simulink model "CarSim_SCANeR_UDP_LKA_THESIS"  (R2019a)
settings: Solver=FixedStepDiscrete  StartTime=0.0  StopTime=inf  FixedStep=0.001  RelTol=1e-3  EnableMultiTasking=on
undefined symbols (not defined in the file or in its folder): DiscIntNeverNeededParam
libraries: simulink x11, xpcutilitieslib x2, xpcrtudplib x2, dspnetwork x1
(part 1 of 2)
settings Model: ExtModeTrigDuration=10000  Creator=llacroix  LastModifiedBy=wilkerson.102
settings SolverCC: PositivePriorityOrder=on  InsertRTBMode=Always
settings DataIOCC: ReturnWorkspaceOutputs=off
settings OptimizationCC: UseFloatMulNetSlope=on
settings DebuggingCC: ArithmeticOperatorsInVariantConditions=warning
settings SFSimCC: SimUseLocalCustomCode=off
settings RTWCC: Description=Generic Real-Time Target  RTWUseLocalCustomCode=off  TargetLang=C++
settings CodeAppCC: StateflowObjectComments=on
settings GRTTargetCC: TargetLangStandard=C++03 (ISO)  MatFileLogging=off  MultiInstanceERTCode=on  CodeInterfacePackaging=C++ class

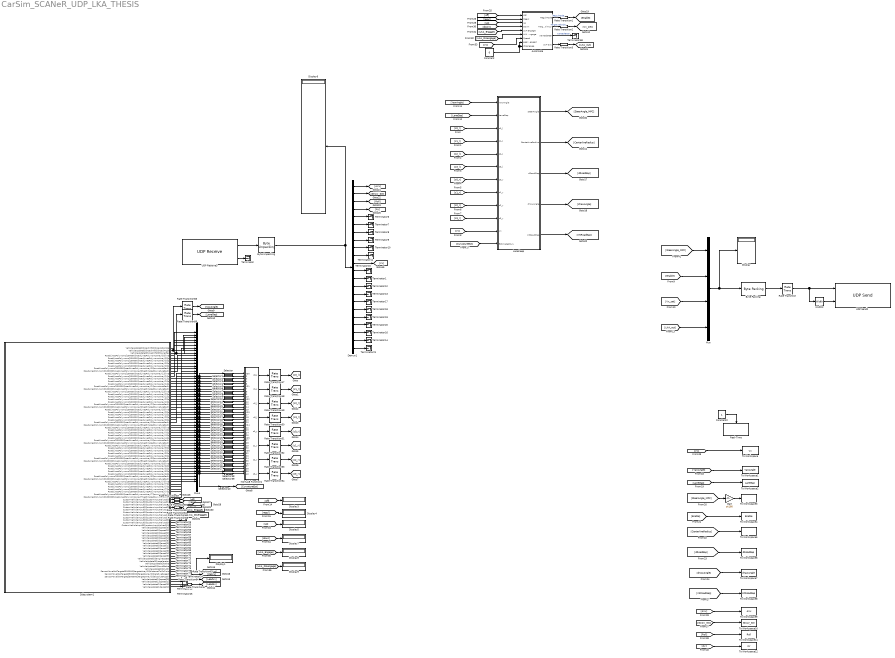
== system CarSim_SCANeR_UDP_LKA_THESIS ==
  Automate : Subsystem
  "Byte Packing " : xpcutilitieslib/Byte Packing   MaskPackedDataType=uint8  MaskUnpackedDataTypes={'double'}  MaskAlignment=1
  "Byte Unpacking " : xpcutilitieslib/Byte Unpacking   MaskUnpackedDataTypes={'double'}  MaskUnpackedDataSizes={[22]}  MaskAlignment=1
      settings: SourceProductName=Simulink Real-Time  SourceProductBaseCode=XP
  Constant : Constant  Value=0
  Constant2 : Constant
  Demux1 : Demux  Outputs=22
  Display{,1,3..9} (9 alike) : Display
  Gain : Gain  Gain=pi/180
  LaneKeep : Subsystem
  MATLAB Function1 : Subsystem
      mask help: Simulink:masks:GenSFuncDesc_MD
      mask Help: eval('feval(''rtwprivate'',''rtwhelpview'',''rtw_sfcn_block'')');
  Mux : Mux
  Mux4 : Mux  Inputs=59
  Rate Transition{,1..3,5,47..64} (23 alike) : RateTransition
  Real-Time : Subsystem
  Selector : Selector  InputPortWidth=59  IndexOptions=Index vector (dialog)  Indices=4  OutputSizes=1
  Selector1 : Selector  InputPortWidth=59  IndexOptions=Index vector (dialog)  Indices=5  OutputSizes=1
  Selector10 : Selector  InputPortWidth=59  IndexOptions=Index vector (dialog)  Indices=18  OutputSizes=1
  Selector11 : Selector  InputPortWidth=59  IndexOptions=Index vector (dialog)  Indices=19  OutputSizes=1
  Selector12 : Selector  InputPortWidth=59  IndexOptions=Index vector (dialog)  Indices=20  OutputSizes=1
  Selector13 : Selector  InputPortWidth=59  IndexOptions=Index vector (dialog)  Indices=21  OutputSizes=1
  Selector14 : Selector  InputPortWidth=59  IndexOptions=Index vector (dialog)  Indices=22  OutputSizes=1
  Selector15 : Selector  InputPortWidth=59  IndexOptions=Index vector (dialog)  Indices=25  OutputSizes=1
  Selector16 : Selector  InputPortWidth=59  IndexOptions=Index vector (dialog)  Indices=26  OutputSizes=1
  Selector17 : Selector  InputPortWidth=59  IndexOptions=Index vector (dialog)  Indices=27  OutputSizes=1
  Selector18 : Selector  InputPortWidth=59  IndexOptions=Index vector (dialog)  Indices=28  OutputSizes=1
  Selector19 : Selector  InputPortWidth=59  IndexOptions=Index vector (dialog)  Indices=29  OutputSizes=1
  Selector2 : Selector  InputPortWidth=59  IndexOptions=Index vector (dialog)  Indices=6  OutputSizes=1
  Selector20 : Selector  InputPortWidth=59  IndexOptions=Index vector (dialog)  Indices=32  OutputSizes=1
  Selector21 : Selector  InputPortWidth=59  IndexOptions=Index vector (dialog)  Indices=33  OutputSizes=1
  Selector22 : Selector  InputPortWidth=59  IndexOptions=Index vector (dialog)  Indices=34  OutputSizes=1
  Selector23 : Selector  InputPortWidth=59  IndexOptions=Index vector (dialog)  Indices=35  OutputSizes=1
  Selector24 : Selector  InputPortWidth=59  IndexOptions=Index vector (dialog)  Indices=36  OutputSizes=1
  Selector25 : Selector  InputPortWidth=59  IndexOptions=Index vector (dialog)  Indices=39  OutputSizes=1
  Selector26 : Selector  InputPortWidth=59  IndexOptions=Index vector (dialog)  Indices=40  OutputSizes=1
  Selector27 : Selector  InputPortWidth=59  IndexOptions=Index vector (dialog)  Indices=41  OutputSizes=1
  Selector28 : Selector  InputPortWidth=59  IndexOptions=Index vector (dialog)  Indices=42  OutputSizes=1
  Selector29 : Selector  InputPortWidth=59  IndexOptions=Index vector (dialog)  Indices=43  OutputSizes=1
  Selector3 : Selector  InputPortWidth=59  IndexOptions=Index vector (dialog)  Indices=7  OutputSizes=1
  Selector30 : Selector  InputPortWidth=59  IndexOptions=Index vector (dialog)  Indices=46  OutputSizes=1
  Selector31 : Selector  InputPortWidth=59  IndexOptions=Index vector (dialog)  Indices=47  OutputSizes=1
  Selector32 : Selector  InputPortWidth=59  IndexOptions=Index vector (dialog)  Indices=48  OutputSizes=1
  Selector33 : Selector  InputPortWidth=59  IndexOptions=Index vector (dialog)  Indices=49  OutputSizes=1
  Selector34 : Selector  InputPortWidth=59  IndexOptions=Index vector (dialog)  Indices=50  OutputSizes=1
  Selector35 : Selector  InputPortWidth=59  IndexOptions=Index vector (dialog)  Indices=53  OutputSizes=1
  Selector36 : Selector  InputPortWidth=59  IndexOptions=Index vector (dialog)  Indices=54  OutputSizes=1
  Selector37 : Selector  InputPortWidth=59  IndexOptions=Index vector (dialog)  Indices=55  OutputSizes=1
  Selector38 : Selector  InputPortWidth=59  IndexOptions=Index vector (dialog)  Indices=56  OutputSizes=1
  Selector39 : Selector  InputPortWidth=59  IndexOptions=Index vector (dialog)  Indices=57  OutputSizes=1
  Selector4 : Selector  InputPortWidth=59  IndexOptions=Index vector (dialog)  Indices=8  OutputSizes=1
  Selector40 : Selector  InputPortWidth=59  IndexOptions=Index vector (dialog)  Indices=10  OutputSizes=1
  Selector5 : Selector  InputPortWidth=59  IndexOptions=Index vector (dialog)  Indices=11  OutputSizes=1
  Selector6 : Selector  InputPortWidth=59  IndexOptions=Index vector (dialog)  Indices=12  OutputSizes=1
  Selector7 : Selector  InputPortWidth=59  IndexOptions=Index vector (dialog)  Indices=13  OutputSizes=1
  Selector8 : Selector  InputPortWidth=59  IndexOptions=Index vector (dialog)  Indices=14  OutputSizes=1
  Selector9 : Selector  InputPortWidth=59  IndexOptions=Index vector (dialog)  Indices=15  OutputSizes=1
  Subsystem1 : Subsystem
  Terminator{,1,6..25,53..63,68..78} (44 alike) : Terminator
  To Workspace : ToWorkspace  VariableName=Vx  SampleTime=-1
      settings: Save2DSignal=2-D array (concatenate along first dimension)
  To Workspace1 : ToWorkspace  VariableName=YawAngle  SampleTime=-1
      settings: Save2DSignal=2-D array (concatenate along first dimension)
  To Workspace10 : ToWorkspace  VariableName=StrAV_SW  SampleTime=-1
      settings: Save2DSignal=2-D array (concatenate along first dimension)
  To Workspace11 : ToWorkspace  VariableName=Roll  SampleTime=-1
      settings: Save2DSignal=2-D array (concatenate along first dimension)
  To Workspace12 : ToWorkspace  VariableName=Ay  SampleTime=-1
      settings: Save2DSignal=2-D array (concatenate along first dimension)
  To Workspace2 : ToWorkspace  VariableName=LaneGap  SampleTime=-1
      settings: Save2DSignal=2-D array (concatenate along first dimension)
  To Workspace3 : ToWorkspace  VariableName=SteerAngle_MPC  SampleTime=-1
      settings: Save2DSignal=2-D array (concatenate along first dimension)
  To Workspace4 : ToWorkspace  VariableName=Enable  SampleTime=-1
      settings: Save2DSignal=2-D array (concatenate along first dimension)
  To Workspace5 : ToWorkspace  VariableName=CenterlineRadius  SampleTime=-1
      settings: Save2DSignal=2-D array (concatenate along first dimension)
  To Workspace6 : ToWorkspace  VariableName=dRoadGap  SampleTime=-1
      settings: Save2DSignal=2-D array (concatenate along first dimension)
  To Workspace7 : ToWorkspace  VariableName=dYawAngle  SampleTime=-1
      settings: Save2DSignal=2-D array (concatenate along first dimension)
  To Workspace8 : ToWorkspace  VariableName=intRoadGap  SampleTime=-1
      settings: Save2DSignal=2-D array (concatenate along first dimension)
  To Workspace9 : ToWorkspace  VariableName=AVx  SampleTime=-1
      settings: Save2DSignal=2-D array (concatenate along first dimension)
  UDP Receive3 : xpcrtudplib/UDP Receive  ipAddressVal=Use host-target connection  localPort=25002  rcvWidth=176  rcvFmAny=off  fmAddress=0.0.0.0  rcvMulticast=off  multicastAddress={}  maxUDPQueue=8  sampleTime=0.001
      settings: SourceProductName=Simulink Real-Time
  UDP Send2 : xpcrtudplib/UDP Send  ipAddressVal=Use host-target connection  localPort=-1  toAddress=255.255.255.255  toPort=25003  sampleTime=0.01
      settings: SourceProductName=Simulink Real-Time  SourceProductBaseCode=XP
  Width2 : Width
  wires:
  Width2/1 -> UDP Send2/2
  UDP Receive3/1 -> "Byte Unpacking "/1
  UDP Receive3/2 -> Terminator/1
  LaneKeep/1(SteerAngle) -> [SteerAngle_MPC]
  [YawAngle] -> LaneKeep/1(YawAngle)
  [LaneGap] -> LaneKeep/2(LaneGap)
  [c0_l] -> LaneKeep/3(c0_l)
  [c1_l] -> LaneKeep/4(c1_l)
  [c2_l] -> LaneKeep/5(c2_l)
  [c3_l] -> LaneKeep/6(c3_l)
  [c0_r] -> LaneKeep/7(c0_r)
  [c1_r] -> LaneKeep/8(c1_r)
  [c2_r] -> LaneKeep/9(c2_r)
  [c3_r] -> LaneKeep/10(c3_r)
  [Vx] -> LaneKeep/11(Vx)
  Demux1/11 -> [Vx]
  Demux1/13 -> Terminator1/1
  [SteerAngle_MPC] -> Mux/1
  "Byte Unpacking "/1 -> Demux1/1, Display6/1
  Mux/1 -> "Byte Packing "/1, Display/1
  "Byte Packing "/1 -> Rate Transition/1
  Rate Transition64/1 -> [RelVx]
  Rate Transition63/1 -> Display1/1, [RelDist]
  Rate Transition58/1 -> [LKA_Disengage]
  Subsystem1/65(CustomVehicleInput[0]/customInputValues[5]) -> Rate Transition58/1
  Rate Transition62/1 -> [LKA_Engage]
  Subsystem1/64(CustomVehicleInput[0]/customInputValues[4]) -> Rate Transition62/1
  Rate Transition61/1 -> [down]
  Subsystem1/63(CustomVehicleInput[0]/customInputValues[3]) -> Rate Transition61/1
  Rate Transition60/1 -> [up]
  Subsystem1/62(CustomVehicleInput[0]/customInputValues[2]) -> Rate Transition60/1
  Rate Transition59/1 -> [regul]
  Subsystem1/61(CustomVehicleInput[0]/customInputValues[1]) -> Rate Transition59/1
  Subsystem1/60(CustomVehicleInput[0]/customInputValues[0]) -> Rate Transition57/1
  Rate Transition57/1 -> [off]
  Rate Transition56/1 -> [LaneGap]
  Rate Transition55/1 -> [YawAngle]
  Rate Transition54/1 -> [c3_r]
  Rate Transition53/1 -> [c2_r]
  Rate Transition52/1 -> [c1_r]
  Rate Transition51/1 -> [c0_r]
  Rate Transition50/1 -> [c3_l]
  Rate Transition49/1 -> [c2_l]
  Rate Transition48/1 -> [c1_l]
  Rate Transition47/1 -> [c0_l]
  Subsystem1/87(VehicleUpdate[0]/clutch) -> Terminator78/1
  Subsystem1/86(VehicleUpdate[0]/handBrake) -> Terminator77/1
  Subsystem1/85(VehicleUpdate[0]/brake) -> Terminator76/1
  Subsystem1/84(VehicleUpdate[0]/accelerator) -> Terminator75/1
  Subsystem1/83(VehicleUpdate[0]/engineSpeed) -> Terminator74/1
  Subsystem1/82(VehicleUpdate[0]/accel[5]) -> Terminator73/1
  Subsystem1/81(VehicleUpdate[0]/accel[4]) -> Terminator72/1
  Subsystem1/80(VehicleUpdate[0]/accel[3]) -> Terminator71/1
  Subsystem1/79(VehicleUpdate[0]/accel[2]) -> Terminator70/1
  Subsystem1/78(VehicleUpdate[0]/accel[1]) -> Terminator69/1
  Subsystem1/77(VehicleUpdate[0]/accel[0]) -> Terminator63/1
  Subsystem1/76(VehicleUpdate[0]/speed[5]) -> Terminator62/1
  Subsystem1/75(VehicleUpdate[0]/speed[4]) -> Terminator61/1
  Subsystem1/74(VehicleUpdate[0]/speed[3]) -> Terminator60/1
  Subsystem1/73(VehicleUpdate[0]/speed[2]) -> Terminator59/1
  Subsystem1/72(VehicleUpdate[0]/speed[1]) -> Terminator58/1
  Subsystem1/71(VehicleUpdate[0]/speed[0]) -> Terminator57/1
  Subsystem1/70(CustomVehicleInput[0]/customInputValues[10]) -> Terminator56/1
  Subsystem1/69(CustomVehicleInput[0]/customInputValues[9]) -> Terminator55/1
  Subsystem1/68(CustomVehicleInput[0]/customInputValues[8]) -> Terminator54/1
  Subsystem1/67(CustomVehicleInput[0]/customInputValues[7]) -> Terminator53/1
  Subsystem1/66(CustomVehicleInput[0]/customInputValues[6]) -> Terminator23/1
  Subsystem1/59(RoadLinesPolynoms[100000]/roadLinesPolynomsArray[7]/estimatedCurvatureRadius) -> Mux4/59
  Subsystem1/58(RoadLinesPolynoms[100000]/roadLinesPolynomsArray[7]/curvatureRadius) -> Mux4/58
  Subsystem1/57(RoadLinesPolynoms[100000]/roadLinesPolynomsArray[7]/c3) -> Mux4/57
  Subsystem1/56(RoadLinesPolynoms[100000]/roadLinesPolynomsArray[7]/c2) -> Mux4/56
  Subsystem1/55(RoadLinesPolynoms[100000]/roadLinesPolynomsArray[7]/c1) -> Mux4/55
  Subsystem1/54(RoadLinesPolynoms[100000]/roadLinesPolynomsArray[7]/c0) -> Mux4/54
  Subsystem1/53(RoadLinesPolynoms[100000]/roadLinesPolynomsArray[7]/lineId) -> Mux4/53
  Subsystem1/52(RoadLinesPolynoms[100000]/roadLinesPolynomsArray[6]/estimatedCurvatureRadius) -> Mux4/52
  Subsystem1/51(RoadLinesPolynoms[100000]/roadLinesPolynomsArray[6]/curvatureRadius) -> Mux4/51
  Subsystem1/50(RoadLinesPolynoms[100000]/roadLinesPolynomsArray[6]/c3) -> Mux4/50
  Subsystem1/49(RoadLinesPolynoms[100000]/roadLinesPolynomsArray[6]/c2) -> Mux4/49
  Subsystem1/48(RoadLinesPolynoms[100000]/roadLinesPolynomsArray[6]/c1) -> Mux4/48
  Subsystem1/47(RoadLinesPolynoms[100000]/roadLinesPolynomsArray[6]/c0) -> Mux4/47
  Subsystem1/46(RoadLinesPolynoms[100000]/roadLinesPolynomsArray[6]/lineId) -> Mux4/46
  Subsystem1/45(RoadLinesPolynoms[100000]/roadLinesPolynomsArray[5]/estimatedCurvatureRadius) -> Mux4/45
  Subsystem1/44(RoadLinesPolynoms[100000]/roadLinesPolynomsArray[5]/curvatureRadius) -> Mux4/44
  Subsystem1/43(RoadLinesPolynoms[100000]/roadLinesPolynomsArray[5]/c3) -> Mux4/43
  Subsystem1/42(RoadLinesPolynoms[100000]/roadLinesPolynomsArray[5]/c2) -> Mux4/42
  Subsystem1/41(RoadLinesPolynoms[100000]/roadLinesPolynomsArray[5]/c1) -> Mux4/41
  Subsystem1/40(RoadLinesPolynoms[100000]/roadLinesPolynomsArray[5]/c0) -> Mux4/40
  Subsystem1/39(RoadLinesPolynoms[100000]/roadLinesPolynomsArray[5]/lineId) -> Mux4/39
  Subsystem1/38(RoadLinesPolynoms[100000]/roadLinesPolynomsArray[4]/estimatedCurvatureRadius) -> Mux4/38
  Subsystem1/37(RoadLinesPolynoms[100000]/roadLinesPolynomsArray[4]/curvatureRadius) -> Mux4/37
  Subsystem1/36(RoadLinesPolynoms[100000]/roadLinesPolynomsArray[4]/c3) -> Mux4/36
  Subsystem1/35(RoadLinesPolynoms[100000]/roadLinesPolynomsArray[4]/c2) -> Mux4/35
  Subsystem1/34(RoadLinesPolynoms[100000]/roadLinesPolynomsArray[4]/c1) -> Mux4/34
  Subsystem1/33(RoadLinesPolynoms[100000]/roadLinesPolynomsArray[4]/c0) -> Mux4/33
  Subsystem1/32(RoadLinesPolynoms[100000]/roadLinesPolynomsArray[4]/lineId) -> Mux4/32
  Subsystem1/31(RoadLinesPolynoms[100000]/roadLinesPolynomsArray[3]/estimatedCurvatureRadius) -> Mux4/31
  Subsystem1/30(RoadLinesPolynoms[100000]/roadLinesPolynomsArray[3]/curvatureRadius) -> Mux4/30
  Subsystem1/29(RoadLinesPolynoms[100000]/roadLinesPolynomsArray[3]/c3) -> Mux4/29
  Subsystem1/28(RoadLinesPolynoms[100000]/roadLinesPolynomsArray[3]/c2) -> Mux4/28
  Subsystem1/27(RoadLinesPolynoms[100000]/roadLinesPolynomsArray[3]/c1) -> Mux4/27
  Subsystem1/26(RoadLinesPolynoms[100000]/roadLinesPolynomsArray[3]/c0) -> Mux4/26
  Subsystem1/25(RoadLinesPolynoms[100000]/roadLinesPolynomsArray[3]/lineId) -> Mux4/25
  Subsystem1/24(RoadLinesPolynoms[100000]/roadLinesPolynomsArray[2]/estimatedCurvatureRadius) -> Mux4/24
  Subsystem1/23(RoadLinesPolynoms[100000]/roadLinesPolynomsArray[2]/curvatureRadius) -> Mux4/23
  Subsystem1/22(RoadLinesPolynoms[100000]/roadLinesPolynomsArray[2]/c3) -> Mux4/22
  Subsystem1/21(RoadLinesPolynoms[100000]/roadLinesPolynomsArray[2]/c2) -> Mux4/21
  Subsystem1/20(RoadLinesPolynoms[100000]/roadLinesPolynomsArray[2]/c1) -> Mux4/20
  Subsystem1/19(RoadLinesPolynoms[100000]/roadLinesPolynomsArray[2]/c0) -> Mux4/19
  Subsystem1/18(RoadLinesPolynoms[100000]/roadLinesPolynomsArray[2]/lineId) -> Mux4/18
  Subsystem1/17(RoadLinesPolynoms[100000]/roadLinesPolynomsArray[1]/estimatedCurvatureRadius) -> Mux4/17
  Subsystem1/16(RoadLinesPolynoms[100000]/roadLinesPolynomsArray[1]/curvatureRadius) -> Mux4/16
  Subsystem1/15(RoadLinesPolynoms[100000]/roadLinesPolynomsArray[1]/c3) -> Mux4/15
  Subsystem1/14(RoadLinesPolynoms[100000]/roadLinesPolynomsArray[1]/c2) -> Mux4/14
  Subsystem1/13(RoadLinesPolynoms[100000]/roadLinesPolynomsArray[1]/c1) -> Mux4/13
  Subsystem1/12(RoadLinesPolynoms[100000]/roadLinesPolynomsArray[1]/c0) -> Mux4/12
  Subsystem1/11(RoadLinesPolynoms[100000]/roadLinesPolynomsArray[1]/lineId) -> Mux4/11
  Subsystem1/10(RoadLinesPolynoms[100000]/roadLinesPolynomsArray[0]/estimatedCurvatureRadius) -> Mux4/10
  Subsystem1/9(RoadLinesPolynoms[100000]/roadLinesPolynomsArray[0]/curvatureRadius) -> Mux4/9
  Subsystem1/8(RoadLinesPolynoms[100000]/roadLinesPolynomsArray[0]/c3) -> Mux4/8
  Subsystem1/7(RoadLinesPolynoms[100000]/roadLinesPolynomsArray[0]/c2) -> Mux4/7
  Subsystem1/6(RoadLinesPolynoms[100000]/roadLinesPolynomsArray[0]/c1) -> Mux4/6
  Subsystem1/5(RoadLinesPolynoms[100000]/roadLinesPolynomsArray[0]/c0) -> Mux4/5
  Subsystem1/4(RoadLinesPolynoms[100000]/roadLinesPolynomsArray[0]/lineId) -> Mux4/4
  Subsystem1/3(VehicleUpdate[0]/roadInfo[0]/laneGap) -> Mux4/3, Rate Transition56/1
  Subsystem1/2(VehicleUpdate[0]/roadInfo[0]/roadAngle) -> Mux4/2, Rate Transition55/1
  Subsystem1/1(VehicleUpdate[0]/roadInfo[0]/roadAbscissa) -> Mux4/1
  Selector39/1 -> MATLAB Function1/40(c3_7)
  Selector38/1 -> MATLAB Function1/39(c2_7)
  Selector37/1 -> MATLAB Function1/38(c1_7)
  Selector36/1 -> MATLAB Function1/37(c0_7)
  Selector35/1 -> MATLAB Function1/36(ID7)
  Selector34/1 -> MATLAB Function1/35(c3_6)
  Selector33/1 -> MATLAB Function1/34(c2_6)
  Selector32/1 -> MATLAB Function1/33(c1_6)
  Selector31/1 -> MATLAB Function1/32(c0_6)
  Selector30/1 -> MATLAB Function1/31(ID6)
  Selector29/1 -> MATLAB Function1/30(c3_5)
  Selector28/1 -> MATLAB Function1/29(c2_5)
  Selector27/1 -> MATLAB Function1/28(c1_5)
  Selector26/1 -> MATLAB Function1/27(c0_5)
  Selector25/1 -> MATLAB Function1/26(ID5)
  Selector24/1 -> MATLAB Function1/25(c3_4)
  Selector23/1 -> MATLAB Function1/24(c2_4)
  Selector22/1 -> MATLAB Function1/23(c1_4)
  Selector21/1 -> MATLAB Function1/22(c0_4)
  Selector20/1 -> MATLAB Function1/21(ID4)
  Selector19/1 -> MATLAB Function1/20(c3_3)
  Selector18/1 -> MATLAB Function1/19(c2_3)
  Selector17/1 -> MATLAB Function1/18(c1_3)
  Selector16/1 -> MATLAB Function1/17(c0_3)
  Selector15/1 -> MATLAB Function1/16(ID3)
  Selector14/1 -> MATLAB Function1/15(c3_2)
  Selector13/1 -> MATLAB Function1/14(c2_2)
  Selector12/1 -> MATLAB Function1/13(c1_2)
  Selector11/1 -> MATLAB Function1/12(c0_2)
  Selector10/1 -> MATLAB Function1/11(ID2)
  Selector9/1 -> MATLAB Function1/10(c3_1)
  Selector8/1 -> MATLAB Function1/9(c2_1)
  Selector7/1 -> MATLAB Function1/8(c1_1)
  Selector6/1 -> MATLAB Function1/7(c0_1)
  Selector5/1 -> MATLAB Function1/6(ID1)
  Selector4/1 -> MATLAB Function1/5(c3_0)
  Selector3/1 -> MATLAB Function1/4(c2_0)
  Selector2/1 -> MATLAB Function1/3(c1_0)
  Selector1/1 -> MATLAB Function1/2(c0_0)
  Selector/1 -> MATLAB Function1/1(ID0)
  MATLAB Function1/8(c3_r) -> Rate Transition54/1
  MATLAB Function1/7(c2_r) -> Rate Transition53/1
  MATLAB Function1/6(c1_r) -> Rate Transition52/1
  MATLAB Function1/5(c0_r) -> Rate Transition51/1
  MATLAB Function1/4(c3_l) -> Rate Transition50/1
  MATLAB Function1/3(c2_l) -> Rate Transition49/1
  MATLAB Function1/2(c1_l) -> Rate Transition48/1
  MATLAB Function1/1(c0_l) -> Rate Transition47/1
  Mux4/1 -> Selector40/1, Selector39/1, Selector38/1, Selector37/1, Selector36/1, Selector35/1, Selector34/1, Selector33/1, Selector32/1, Selector31/1, Selector30/1, Selector29/1, Selector28/1, Selector27/1, Selector26/1, Selector25/1, Selector24/1, Selector23/1, Selector22/1, Selector21/1, Selector20/1, Selector19/1, Selector18/1, Selector17/1, Selector16/1, Selector15/1, Selector14/1, Selector11/1, Selector10/1, Selector9/1, Selector7/1, Selector6/1, Selector5/1, Selector4/1, Selector3/1, Selector2/1, Selector/1, Selector1/1, Selector8/1, Selector12/1, Selector13/1
  Subsystem1/89(SensorMovableTargets[300000]/targetsArray[0]/relativeSpeedX) -> Rate Transition64/1
  Subsystem1/88(SensorMovableTargets[300000]/targetsArray[0]/distanceToCollision) -> Rate Transition63/1
  Demux1/3 -> [Roll]
  Demux1/5 -> Terminator6/1
  Demux1/6 -> Terminator7/1
  Demux1/7 -> Terminator8/1
  Demux1/8 -> Terminator9/1
  Demux1/9 -> Terminator10/1
  Demux1/10 -> Terminator11/1
  Demux1/14 -> Terminator12/1
  Demux1/15 -> Terminator13/1
  Demux1/21 -> Terminator14/1
  Automate/2(Target (m/s)) -> Rate Transition2/1  "Target Velocity"
  Automate/1(RegulMode) -> Rate Transition1/1  "RegulMode"
  Automate/3(wantedGear) -> Terminator68/1  "wantedGear"
  Demux1/12 -> Terminator15/1
  Demux1/20 -> Terminator16/1
  Automate/4(LKA Out) -> Rate Transition3/1
  Rate Transition1/1 -> [Enable]
  Rate Transition2/1 -> [Vx_set]
  Rate Transition3/1 -> [LKA_out]
  [off] -> Automate/1(Off)
  [regul] -> Automate/2(Regul)
  [up] -> Automate/3(Up)
  [down] -> Automate/4(Down)
  [LKA_Engage] -> Automate/5(LKA Engage)
  [LKA_Disengage] -> Automate/6(LKA Disengage)
  [Vx] -> Automate/7(Speed)
  Constant/1 -> Automate/9(disengage), Automate/8(gearEngaged)
  Rate Transition/1 -> Width2/1, UDP Send2/1
  [Enable] -> Mux/2
  [Vx_set] -> Mux/3
  [LKA_out] -> Mux/4
  [off] -> Display3/1
  [regul] -> Display4/1
  [up] -> Display5/1
  [down] -> Display7/1
  [LKA_Engage] -> Display8/1
  [LKA_Disengage] -> Display9/1
  Demux1/16 -> Terminator17/1
  Demux1/17 -> Terminator18/1
  Demux1/18 -> Terminator19/1
  Demux1/19 -> Terminator20/1
  Demux1/22 -> Terminator21/1
  Selector40/1 -> [CurvatureEst]
  [CurvatureEst] -> LaneKeep/12(EstimatedCurv)
  Rate Transition5/1 -> [LeadAx]
  Subsystem1/91(VehicleUpdate[1]/speed[0]) -> [LeadVx]
  Subsystem1/93(VehicleUpdate[1]/accel[0]) -> Rate Transition5/1
  Subsystem1/94(VehicleUpdate[1]/accel[1]) -> Terminator25/1
  Subsystem1/92(VehicleUpdate[1]/speed[1]) -> Terminator22/1
  Subsystem1/90(SensorMovableTargets[300000]/targetsArray[0]/absoluteAccelX) -> Terminator24/1
  Constant2/1 -> Real-Time/Enable
  [Vx] -> To Workspace/1
  LaneKeep/2(CenterLineRadius) -> [CenterlineRadius]
  [SteerAngle_MPC] -> Gain/1
  LaneKeep/3(dRoadGap) -> [dRoadGap]
  LaneKeep/4(dYawAngle) -> [dYawAngle]
  LaneKeep/5(intRoadGap) -> [intRoadGap]
  [YawAngle] -> To Workspace1/1
  [LaneGap] -> To Workspace2/1
  Gain/1 -> To Workspace3/1
  [Enable] -> To Workspace4/1
  [CenterlineRadius] -> To Workspace5/1
  [dRoadGap] -> To Workspace6/1
  [dYawAngle] -> To Workspace7/1
  [intRoadGap] -> To Workspace8/1
  Demux1/1 -> [AVx]
  Demux1/2 -> [StrAV_SW]
  [AVx] -> To Workspace9/1
  [StrAV_SW] -> To Workspace10/1
  [Roll] -> To Workspace11/1
  Demux1/4 -> [Ay]
  [Ay] -> To Workspace12/1

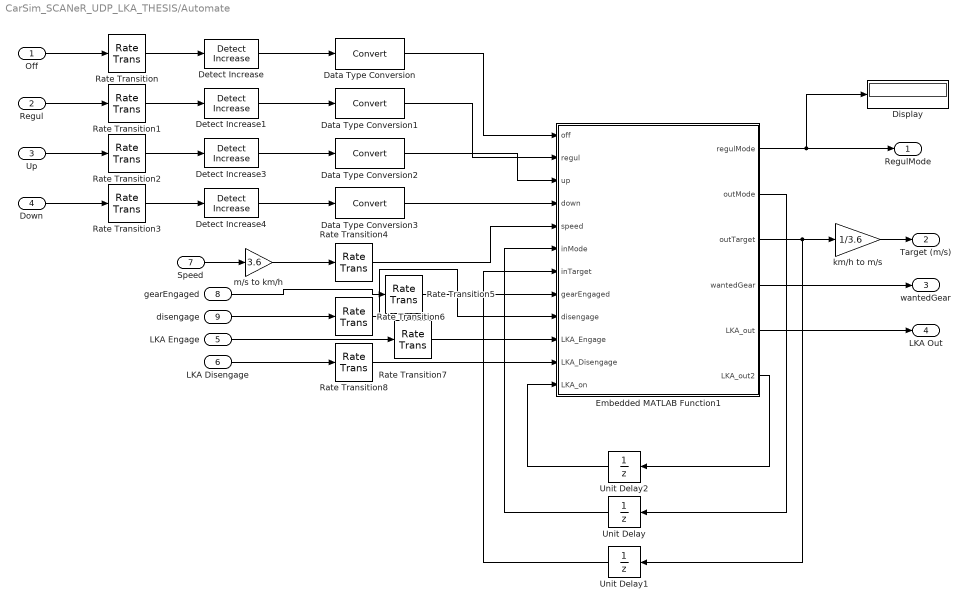
== system CarSim_SCANeR_UDP_LKA_THESIS/Automate ==
  Off : Inport  PortDimensions=1
  Regul : Inport  Port=2  PortDimensions=1
  Up : Inport  Port=3  PortDimensions=1
  Down : Inport  Port=4  PortDimensions=1
  LKA Engage : Inport  Port=5  PortDimensions=1
  LKA Disengage : Inport  Port=6  PortDimensions=1
  Speed : Inport  Port=7  PortDimensions=1
  gearEngaged : Inport  Port=8  PortDimensions=1
  disengage : Inport  Port=9  PortDimensions=1
  Data Type Conversion{,1..3} (4 alike) : DataTypeConversion
  Detect Increase{,1,3..4} (4 alike) : simulink/Logic and Bit Operations/Detect Increase  vinit=0.0  OutDataTypeStr=uint8
  Display : Display
  Embedded MATLAB Function1 : MATLAB Function  TreatAsAtomicUnit=on
  Rate Transition{,1..8} (9 alike) : RateTransition
  Unit Delay : UnitDelay  SampleTime=-1
  Unit Delay1 : UnitDelay  SampleTime=-1
  Unit Delay2 : UnitDelay  SampleTime=-1
  km/h to m/s : Gain  Gain=1/3.6
  m/s to km/h : Gain  Gain=3.6
  RegulMode : Outport
  Target (m/s) : Outport  Port=2
  wantedGear : Outport  Port=3
  LKA Out : Outport  Port=4
  wires:
  Rate Transition8/1 -> Embedded MATLAB Function1/11(LKA_Disengage)
  Rate Transition7/1 -> Embedded MATLAB Function1/10(LKA_Engage)
  Rate Transition6/1 -> Embedded MATLAB Function1/9(disengage)
  Rate Transition5/1 -> Embedded MATLAB Function1/8(gearEngaged)
  Rate Transition4/1 -> Embedded MATLAB Function1/5(speed)
  Rate Transition3/1 -> Detect Increase4/1
  Rate Transition2/1 -> Detect Increase3/1
  Rate Transition1/1 -> Detect Increase1/1
  Rate Transition/1 -> Detect Increase/1
  Data Type Conversion3/1 -> Embedded MATLAB Function1/4(down)
  Data Type Conversion2/1 -> Embedded MATLAB Function1/3(up)
  Data Type Conversion1/1 -> Embedded MATLAB Function1/2(regul)
  Data Type Conversion/1 -> Embedded MATLAB Function1/1(off)
  Unit Delay2/1 -> Embedded MATLAB Function1/12(LKA_on)
  Embedded MATLAB Function1/6(LKA_out2) -> Unit Delay2/1
  disengage/1 -> Rate Transition6/1
  gearEngaged/1 -> Rate Transition5/1
  Speed/1 -> m/s to km/h/1
  LKA Disengage/1 -> Rate Transition8/1
  LKA Engage/1 -> Rate Transition7/1
  Embedded MATLAB Function1/5(LKA_out) -> LKA Out/1
  Off/1 -> Rate Transition/1
  Down/1 -> Rate Transition3/1
  Up/1 -> Rate Transition2/1
  Regul/1 -> Rate Transition1/1
  km/h to m/s/1 -> Target (m/s)/1
  Detect Increase/1 -> Data Type Conversion/1
  Detect Increase1/1 -> Data Type Conversion1/1
  Detect Increase3/1 -> Data Type Conversion2/1
  Detect Increase4/1 -> Data Type Conversion3/1
  m/s to km/h/1 -> Rate Transition4/1
  Embedded MATLAB Function1/4(wantedGear) -> wantedGear/1
  Embedded MATLAB Function1/3(outTarget) -> km/h to m/s/1, Unit Delay1/1
  Unit Delay/1 -> Embedded MATLAB Function1/6(inMode)
  Embedded MATLAB Function1/2(outMode) -> Unit Delay/1
  Unit Delay1/1 -> Embedded MATLAB Function1/7(inTarget)
  Embedded MATLAB Function1/1(regulMode) -> Display/1, RegulMode/1

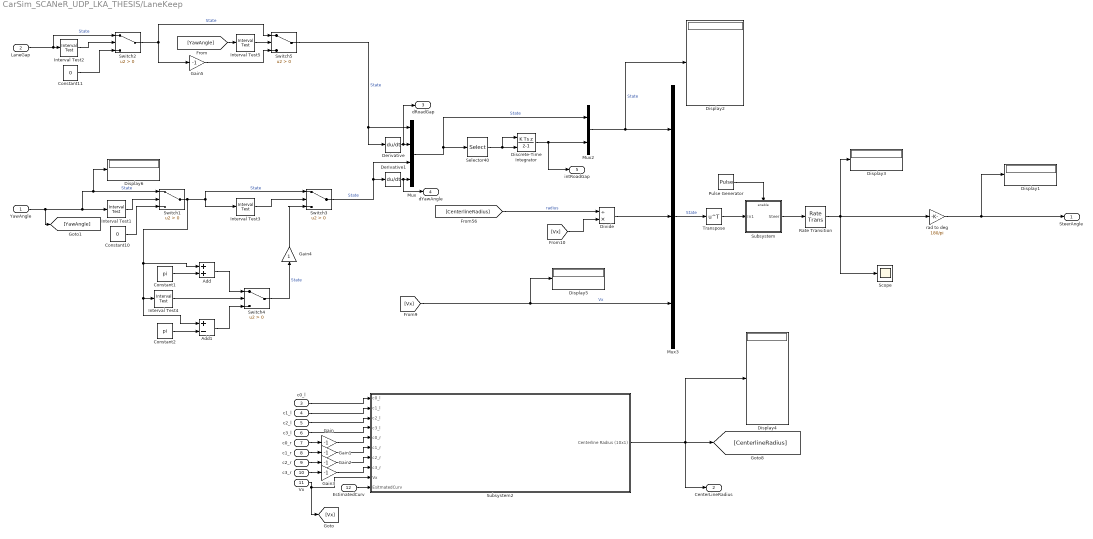
== system CarSim_SCANeR_UDP_LKA_THESIS/LaneKeep ==
  YawAngle : Inport
  LaneGap : Inport  Port=2
  c0_l : Inport  Port=3
  c1_l : Inport  Port=4
  c2_l : Inport  Port=5
  c3_l : Inport  Port=6
  c0_r : Inport  Port=7
  c1_r : Inport  Port=8
  c2_r : Inport  Port=9
  c3_r : Inport  Port=10
  Vx : Inport  Port=11
  EstimatedCurv : Inport  Port=12
  Add : Sum
  Add1 : Sum  Inputs=+-
  Constant1 : Constant  Value=pi
  Constant10 : Constant  Value=0
  Constant11 : Constant  Value=0
  Constant2 : Constant  Value=pi
  Derivative : Derivative
  Derivative1 : Derivative
  Discrete-Time Integrator : DiscreteIntegrator  IntegratorMethod=Integration: Backward Euler  ExternalReset=either  SampleTime=-1  ICPrevOutput=DiscIntNeverNeededParam  ICPrevScaledInput=DiscIntNeverNeededParam
  Display{1..6} (6 alike) : Display
  Divide : Product  Inputs=/*
  Gain{,1..3,5} (5 alike) : Gain  Gain=-1
  Gain4 : Gain
  Interval Test1 : simulink/Logic and Bit Operations/Interval Test  IntervalClosedRight=on  uplimit=1000  IntervalClosedLeft=on  lowlimit=-1000  OutDataTypeStr=boolean
  Interval Test2 : simulink/Logic and Bit Operations/Interval Test  IntervalClosedRight=on  uplimit=1000  IntervalClosedLeft=on  lowlimit=-1000  OutDataTypeStr=boolean
  Interval Test3 : simulink/Logic and Bit Operations/Interval Test  IntervalClosedRight=on  uplimit=1  IntervalClosedLeft=on  lowlimit=-1  OutDataTypeStr=boolean
  Interval Test4 : simulink/Logic and Bit Operations/Interval Test  IntervalClosedRight=on  uplimit=0  IntervalClosedLeft=on  lowlimit=-1000  OutDataTypeStr=boolean
  Interval Test5 : simulink/Logic and Bit Operations/Interval Test  IntervalClosedRight=on  uplimit=1.5  IntervalClosedLeft=on  lowlimit=-1.5  OutDataTypeStr=boolean
  Mux : Mux
  Mux2 : Mux  Inputs=2
  Mux3 : Mux  Inputs=3
  Pulse Generator : DiscretePulseGenerator  PulseType=Time based  Period=0.01  PulseWidth=10
  Rate Transition : RateTransition
  Scope : Scope
  Selector40 : Selector  InputPortWidth=4  IndexOptions=Index vector (dialog)  Indices=1  OutputSizes=1
  Subsystem : Subsystem
  Subsystem2 : Subsystem
  Switch{1..5} (5 alike) : Switch  Criteria=u2 > Threshold
  Transpose : Math  Operator=transpose  SaturateOnIntegerOverflow=on
  rad to deg : Gain  Gain=180/pi
  SteerAngle : Outport
  CenterLineRadius : Outport  Port=2
  dRoadGap : Outport  Port=3
  dYawAngle : Outport  Port=4
  intRoadGap : Outport  Port=5
  wires:
  [CenterlineRadius] -> Divide/1  "radius"
  Mux3/1 -> Transpose/1  "State"
  c1_r/1 -> Gain1/1
  Mux2/1 -> Display2/1, Mux3/1  "State"
  Derivative1/1 -> dYawAngle/1, Mux/4
  Interval Test2/1 -> Switch2/2
  Constant11/1 -> Switch2/3
  Derivative/1 -> dRoadGap/1, Mux/2
  [Vx] -> Display5/1, Mux3/3  "Vx"
  Mux/1 -> Mux2/1, Selector40/1  "State"
  c2_r/1 -> Gain2/1
  Switch3/1 -> Derivative1/1, Mux/3  "State"
  YawAngle/1 -> [YawAngle], Display6/1, Switch1/1, Interval Test1/1  "State"
  c0_r/1 -> Gain/1
  Subsystem2/1(Centerline Radius (10x1)) -> Display4/1, CenterLineRadius/1, [CenterlineRadius]
  Interval Test1/1 -> Switch1/2
  c3_r/1 -> Gain3/1
  Switch5/1 -> Derivative/1, Mux/1  "State"
  Selector40/1 -> Discrete-Time Integrator/2, Discrete-Time Integrator/1
  LaneGap/1 -> Interval Test2/1, Switch2/1  "State"
  [Vx] -> Divide/2
  Divide/1 -> Mux3/2
  Constant10/1 -> Switch1/3
  c0_l/1 -> Subsystem2/1(c0_l)
  c1_l/1 -> Subsystem2/2(c1_l)
  c2_l/1 -> Subsystem2/3(c2_l)
  c3_l/1 -> Subsystem2/4(c3_l)
  Gain/1 -> Subsystem2/5(c0_r)
  Gain1/1 -> Subsystem2/6(c1_r)
  Gain2/1 -> Subsystem2/7(c2_r)
  Gain3/1 -> Subsystem2/8(c3_r)
  Vx/1 -> Subsystem2/9(Vx), [Vx]
  rad to deg/1 -> Display1/1, SteerAngle/1
  Interval Test3/1 -> Switch3/2
  Switch1/1 -> Add/1, Add1/1, Interval Test4/1, Interval Test3/1, Switch3/1  "State"
  Interval Test4/1 -> Switch4/2
  Constant1/1 -> Add/2
  Add/1 -> Switch4/1
  Constant2/1 -> Add1/2
  Add1/1 -> Switch4/3
  Switch4/1 -> Gain4/1  "State"
  Gain4/1 -> Switch3/3
  Discrete-Time Integrator/1 -> intRoadGap/1, Mux2/2
  Interval Test5/1 -> Switch5/2
  [YawAngle] -> Interval Test5/1
  Switch2/1 -> Gain5/1, Switch5/1  "State"
  Gain5/1 -> Switch5/3
  EstimatedCurv/1 -> Subsystem2/10(EsitmatedCurv)
  Rate Transition/1 -> Scope/1, Display3/1, rad to deg/1
  Transpose/1 -> Subsystem/1(In1)
  Subsystem/1(Steer) -> Rate Transition/1
  Pulse Generator/1 -> Subsystem/Enable

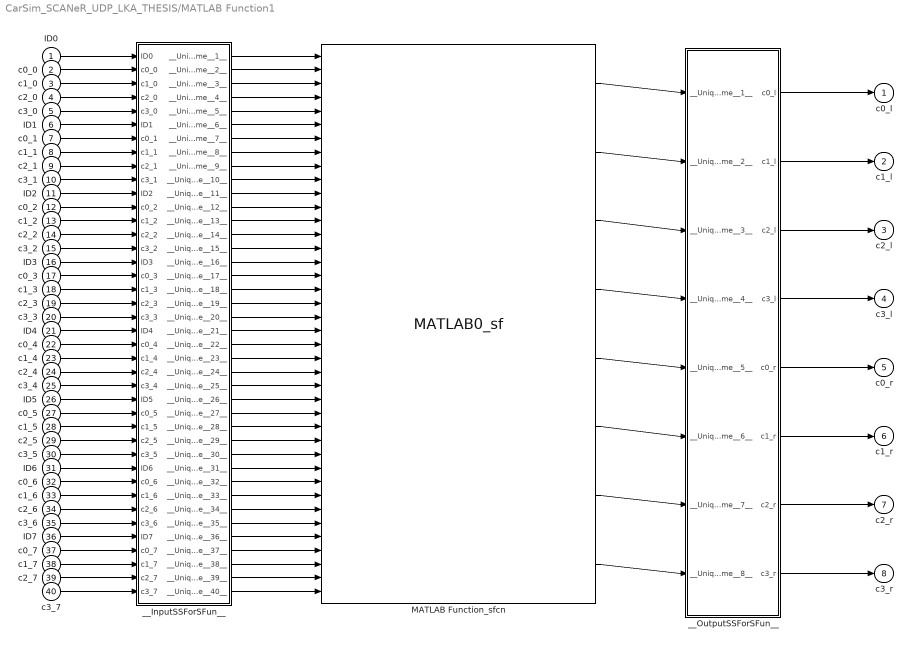
== system CarSim_SCANeR_UDP_LKA_THESIS/MATLAB Function1 ==
  ID0 : Inport
  c0_0 : Inport  Port=2
  c1_0 : Inport  Port=3
  c2_0 : Inport  Port=4
  c3_0 : Inport  Port=5
  ID1 : Inport  Port=6
  c0_1 : Inport  Port=7
  c1_1 : Inport  Port=8
  c2_1 : Inport  Port=9
  c3_1 : Inport  Port=10
  ID2 : Inport  Port=11
  c0_2 : Inport  Port=12
  c1_2 : Inport  Port=13
  c2_2 : Inport  Port=14
  c3_2 : Inport  Port=15
  ID3 : Inport  Port=16
  c0_3 : Inport  Port=17
  c1_3 : Inport  Port=18
  c2_3 : Inport  Port=19
  c3_3 : Inport  Port=20
  ID4 : Inport  Port=21
  c0_4 : Inport  Port=22
  c1_4 : Inport  Port=23
  c2_4 : Inport  Port=24
  c3_4 : Inport  Port=25
  ID5 : Inport  Port=26
  c0_5 : Inport  Port=27
  c1_5 : Inport  Port=28
  c2_5 : Inport  Port=29
  c3_5 : Inport  Port=30
  ID6 : Inport  Port=31
  c0_6 : Inport  Port=32
  c1_6 : Inport  Port=33
  c2_6 : Inport  Port=34
  c3_6 : Inport  Port=35
  ID7 : Inport  Port=36
  c0_7 : Inport  Port=37
  c1_7 : Inport  Port=38
  c2_7 : Inport  Port=39
  c3_7 : Inport  Port=40
  MATLAB Function_sfcn : S-Function  FunctionName=MATLAB0_sf  SFunctionModules=""  SFunctionDeploymentMode=off  EnableBusSupport=off  mask{rtw_sf_name=MATLAB0_sf, showVar=off}
      mask prompts: rtw_sf_name "Simulink:masks:GenSFuncName_MP"; showVar "Simulink:masks:GenSFuncShowModuleList_MP"
      mask help: Simulink:masks:GenSFuncDesc_MD
      mask init:
      | displist = '';
      | if ~strcmp(get_param(gcb, 'FunctionName'), rtw_sf_name);
      |   set_param(gcb, 'FunctionName', rtw_sf_name);
      | end
      | % Check if we are generating code
      | rtw_mode = false;
      | if strcmpi(get_param(bdroot(gcb),'SimulationStatus'),'Initializing')
      | 	rtw_mode = strcmpi(get_param(bdroot(gcb),'BuildingRTWCode'),'on') && ...
      | 		~strcmpi(get_param(bdroot(gcb),'TargetStyle'),'SimulationTarget');
      | end
      | if showVar || rtw_mode
      | 	if exist('rtwsfunc') == 2 | exist('rtwsfunc') == 6
      | 		tmplist = rtwsfunc(rtw_sf_name,gcb);
      | 		tmplist = DAStudio.message('Simulink:masks:GenSFuncListOfModules_IC', tmplist);
      | 	elseif showVar
      | 		tmplist1 = DAStudio.message('Simulink:masks:GenSFuncListOfModules_IC', '');
      |         tmplist2 = DAStudio.message('Simulink:masks:GenSFuncNotLicensed_IC');
      |         tmplist = [tmplist1 tmplist2];
      |  	end
      | end
      | if showVar
      |   displist = tmplist;
      | end
      settings: CopyFcn=|
      | if ~strcmp(get_param(gcb,'Linkstatus'),'none') && ...
      | ~strcmp(get_param(gcb,'Linkstatus'),'implicit')
      |   set_param(gcb,'LinkStatus','none');
      | end
      mask Help: eval('feval(''rtwprivate'',''rtwhelpview'',''rtw_sfcn_block'')');
      mask Display:
      | port_label('input',1,'ID0');
      | port_label('input',2,'c0_0');
      | port_label('input',3,'c1_0');
      | port_label('input',4,'c2_0');
      | port_label('input',5,'c3_0');
      | port_label('input',6,'ID1');
      | port_label('input',7,'c0_1');
      | port_label('input',8,'c1_1');
      | port_label('input',9,'c2_1');
      | port_label('input',10,'c3_1');
      | port_label('input',11,'ID2');
      | port_label('input',12,'c0_2');
      | port_label('input',13,'c1_2');
      | port_label('input',14,'c2_2');
      | port_label('input',15,'c3_2');
      | port_label('input',16,'ID3');
      | port_label('input',17,'c0_3');
      | port_label('input',18,'c1_3');
      | port_label('input',19,'c2_3');
      | port_label('input',20,'c3_3');
      | port_label('input',21,'ID4');
      | port_label('input',22,'c0_4');
      | port_label('input',23,'c1_4');
      | port_label('input',24,'c2_4');
      | port_label('input',25,'c3_4');
      | port_label('input',26,'ID5');
      | port_label('input',27,'c0_5');
      | port_label('input',28,'c1_5');
      | port_label('input',29,'c2_5');
      | port_label('input',30,'c3_5');
      | port_label('input',31,'ID6');
      | port_label('input',32,'c0_6');
      | port_label('input',33,'c1_6');
      | port_label('input',34,'c2_6');
      | port_label('input',35,'c3_6');
      | port_label('input',36,'ID7');
      | port_label('input',37,'c0_7');
      | port_label('input',38,'c1_7');
      | port_label('input',39,'c2_7');
      | port_label('input',40,'c3_7');
      | port_label('output',1,'c0_l');
      | port_label('output',2,'c1_l');
      | port_label('output',3,'c2_l');
      | port_label('output',4,'c3_l');
      | port_label('output',5,'c0_r');
      | port_label('output',6,'c1_r');
      | port_label('output',7,'c2_r');
      | port_label('output',8,'c3_r');
  __InputSSForSFun__ : Subsystem
  __OutputSSForSFun__ : Subsystem
  c0_l : Outport
  c1_l : Outport  Port=2
  c2_l : Outport  Port=3
  c3_l : Outport  Port=4
  c0_r : Outport  Port=5
  c1_r : Outport  Port=6
  c2_r : Outport  Port=7
  c3_r : Outport  Port=8
  wires:
  ID0/1 -> __InputSSForSFun__/1(ID0)
  c0_0/1 -> __InputSSForSFun__/2(c0_0)
  c1_0/1 -> __InputSSForSFun__/3(c1_0)
  c2_0/1 -> __InputSSForSFun__/4(c2_0)
  c3_0/1 -> __InputSSForSFun__/5(c3_0)
  ID1/1 -> __InputSSForSFun__/6(ID1)
  c0_1/1 -> __InputSSForSFun__/7(c0_1)
  c1_1/1 -> __InputSSForSFun__/8(c1_1)
  c2_1/1 -> __InputSSForSFun__/9(c2_1)
  c3_1/1 -> __InputSSForSFun__/10(c3_1)
  ID2/1 -> __InputSSForSFun__/11(ID2)
  c0_2/1 -> __InputSSForSFun__/12(c0_2)
  c1_2/1 -> __InputSSForSFun__/13(c1_2)
  c2_2/1 -> __InputSSForSFun__/14(c2_2)
  c3_2/1 -> __InputSSForSFun__/15(c3_2)
  ID3/1 -> __InputSSForSFun__/16(ID3)
  c0_3/1 -> __InputSSForSFun__/17(c0_3)
  c1_3/1 -> __InputSSForSFun__/18(c1_3)
  c2_3/1 -> __InputSSForSFun__/19(c2_3)
  c3_3/1 -> __InputSSForSFun__/20(c3_3)
  ID4/1 -> __InputSSForSFun__/21(ID4)
  c0_4/1 -> __InputSSForSFun__/22(c0_4)
  c1_4/1 -> __InputSSForSFun__/23(c1_4)
  c2_4/1 -> __InputSSForSFun__/24(c2_4)
  c3_4/1 -> __InputSSForSFun__/25(c3_4)
  ID5/1 -> __InputSSForSFun__/26(ID5)
  c0_5/1 -> __InputSSForSFun__/27(c0_5)
  c1_5/1 -> __InputSSForSFun__/28(c1_5)
  c2_5/1 -> __InputSSForSFun__/29(c2_5)
  c3_5/1 -> __InputSSForSFun__/30(c3_5)
  ID6/1 -> __InputSSForSFun__/31(ID6)
  c0_6/1 -> __InputSSForSFun__/32(c0_6)
  c1_6/1 -> __InputSSForSFun__/33(c1_6)
  c2_6/1 -> __InputSSForSFun__/34(c2_6)
  c3_6/1 -> __InputSSForSFun__/35(c3_6)
  ID7/1 -> __InputSSForSFun__/36(ID7)
  c0_7/1 -> __InputSSForSFun__/37(c0_7)
  c1_7/1 -> __InputSSForSFun__/38(c1_7)
  c2_7/1 -> __InputSSForSFun__/39(c2_7)
  c3_7/1 -> __InputSSForSFun__/40(c3_7)
  __InputSSForSFun__/1(__UniqueOutportName__1__) -> MATLAB Function_sfcn/1
  __InputSSForSFun__/2(__UniqueOutportName__2__) -> MATLAB Function_sfcn/2
  __InputSSForSFun__/3(__UniqueOutportName__3__) -> MATLAB Function_sfcn/3
  __InputSSForSFun__/4(__UniqueOutportName__4__) -> MATLAB Function_sfcn/4
  __InputSSForSFun__/5(__UniqueOutportName__5__) -> MATLAB Function_sfcn/5
  __InputSSForSFun__/6(__UniqueOutportName__6__) -> MATLAB Function_sfcn/6
  __InputSSForSFun__/7(__UniqueOutportName__7__) -> MATLAB Function_sfcn/7
  __InputSSForSFun__/8(__UniqueOutportName__8__) -> MATLAB Function_sfcn/8
  __InputSSForSFun__/9(__UniqueOutportName__9__) -> MATLAB Function_sfcn/9
  __InputSSForSFun__/10(__UniqueOutportName__10__) -> MATLAB Function_sfcn/10
  __InputSSForSFun__/11(__UniqueOutportName__11__) -> MATLAB Function_sfcn/11
  __InputSSForSFun__/12(__UniqueOutportName__12__) -> MATLAB Function_sfcn/12
  __InputSSForSFun__/13(__UniqueOutportName__13__) -> MATLAB Function_sfcn/13
  __InputSSForSFun__/14(__UniqueOutportName__14__) -> MATLAB Function_sfcn/14
  __InputSSForSFun__/15(__UniqueOutportName__15__) -> MATLAB Function_sfcn/15
  __InputSSForSFun__/16(__UniqueOutportName__16__) -> MATLAB Function_sfcn/16
  __InputSSForSFun__/17(__UniqueOutportName__17__) -> MATLAB Function_sfcn/17
  __InputSSForSFun__/18(__UniqueOutportName__18__) -> MATLAB Function_sfcn/18
  __InputSSForSFun__/19(__UniqueOutportName__19__) -> MATLAB Function_sfcn/19
  __InputSSForSFun__/20(__UniqueOutportName__20__) -> MATLAB Function_sfcn/20
  __InputSSForSFun__/21(__UniqueOutportName__21__) -> MATLAB Function_sfcn/21
  __InputSSForSFun__/22(__UniqueOutportName__22__) -> MATLAB Function_sfcn/22
  __InputSSForSFun__/23(__UniqueOutportName__23__) -> MATLAB Function_sfcn/23
  __InputSSForSFun__/24(__UniqueOutportName__24__) -> MATLAB Function_sfcn/24
  __InputSSForSFun__/25(__UniqueOutportName__25__) -> MATLAB Function_sfcn/25
  __InputSSForSFun__/26(__UniqueOutportName__26__) -> MATLAB Function_sfcn/26
  __InputSSForSFun__/27(__UniqueOutportName__27__) -> MATLAB Function_sfcn/27
  __InputSSForSFun__/28(__UniqueOutportName__28__) -> MATLAB Function_sfcn/28
  __InputSSForSFun__/29(__UniqueOutportName__29__) -> MATLAB Function_sfcn/29
  __InputSSForSFun__/30(__UniqueOutportName__30__) -> MATLAB Function_sfcn/30
  __InputSSForSFun__/31(__UniqueOutportName__31__) -> MATLAB Function_sfcn/31
  __InputSSForSFun__/32(__UniqueOutportName__32__) -> MATLAB Function_sfcn/32
  __InputSSForSFun__/33(__UniqueOutportName__33__) -> MATLAB Function_sfcn/33
  __InputSSForSFun__/34(__UniqueOutportName__34__) -> MATLAB Function_sfcn/34
  __InputSSForSFun__/35(__UniqueOutportName__35__) -> MATLAB Function_sfcn/35
  __InputSSForSFun__/36(__UniqueOutportName__36__) -> MATLAB Function_sfcn/36
  __InputSSForSFun__/37(__UniqueOutportName__37__) -> MATLAB Function_sfcn/37
  __InputSSForSFun__/38(__UniqueOutportName__38__) -> MATLAB Function_sfcn/38
  __InputSSForSFun__/39(__UniqueOutportName__39__) -> MATLAB Function_sfcn/39
  __InputSSForSFun__/40(__UniqueOutportName__40__) -> MATLAB Function_sfcn/40
  MATLAB Function_sfcn/1 -> __OutputSSForSFun__/1(__UniqueInportName__1__)
  MATLAB Function_sfcn/2 -> __OutputSSForSFun__/2(__UniqueInportName__2__)
  MATLAB Function_sfcn/3 -> __OutputSSForSFun__/3(__UniqueInportName__3__)
  MATLAB Function_sfcn/4 -> __OutputSSForSFun__/4(__UniqueInportName__4__)
  MATLAB Function_sfcn/5 -> __OutputSSForSFun__/5(__UniqueInportName__5__)
  MATLAB Function_sfcn/6 -> __OutputSSForSFun__/6(__UniqueInportName__6__)
  MATLAB Function_sfcn/7 -> __OutputSSForSFun__/7(__UniqueInportName__7__)
  MATLAB Function_sfcn/8 -> __OutputSSForSFun__/8(__UniqueInportName__8__)
  __OutputSSForSFun__/1(c0_l) -> c0_l/1
  __OutputSSForSFun__/2(c1_l) -> c1_l/1
  __OutputSSForSFun__/3(c2_l) -> c2_l/1
  __OutputSSForSFun__/4(c3_l) -> c3_l/1
  __OutputSSForSFun__/5(c0_r) -> c0_r/1
  __OutputSSForSFun__/6(c1_r) -> c1_r/1
  __OutputSSForSFun__/7(c2_r) -> c2_r/1
  __OutputSSForSFun__/8(c3_r) -> c3_r/1

== system CarSim_SCANeR_UDP_LKA_THESIS/Real-Time ==
  Enable : EnablePort
  Terminator1 : Terminator
  Timer for Real-Time : S-Function  FunctionName=sfun_rttime  Parameters=1  SFunctionDeploymentMode=off  EnableBusSupport=off
  wires:
  Timer for Real-Time/1 -> Terminator1/1
